simulink model "ThreeTankModelIITBombay"  (Simulink 6.6)
settings: Solver=ode3  StartTime=0.0  StopTime=2000  RelTol=1e-3
libraries: simulink3 x4
settings Model: Creator=nina  LastModifiedBy=nina
settings OptimizationCC: InlineInvariantSignals=on
settings DebuggingCC: SignalResolutionControl=TryResolveAllWithWarning  SolverPrmCheckMsg=none  InheritedTsInSrcMsg=none  MultiTaskDSMMsg=warning  MultiTaskCondExecSysMsg=none  StrictBusMsg=None
settings HardwareCC: TargetUnknown=on
settings RTWCC: IncludeERTFirstTime=on
settings STFCustomTargetCC: TargetFcnLib=ansi_tfl_tmw.mat  GenFloatMathFcnCalls=ANSI_C  MatFileLogging=on  SystemTargetFile=grt.tlc

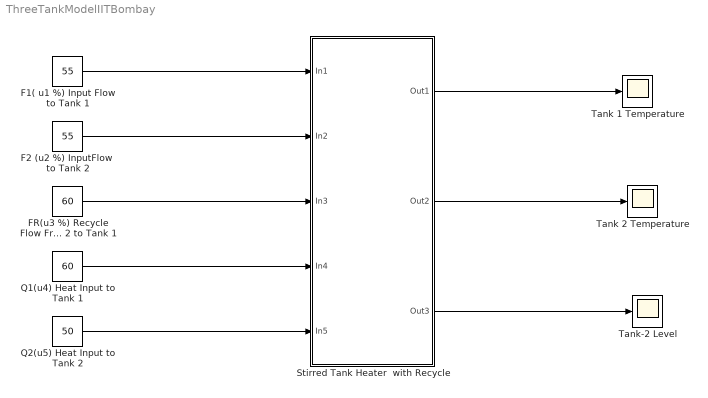
== system ThreeTankModelIITBombay ==
  "F1( u1 %) Input Flow to Tank 1 " : Constant  Value=55
  F2 (u2 %) InputFlow  to Tank 2 : Constant  Value=55
  FR(u3 %) Recycle Flow From Tank 2 to Tank 1 : Constant  Value=60
  Q1(u4) Heat Input to Tank 1 : Constant  Value=60
  Q2(u5) Heat Input to Tank 2 : Constant  Value=50
  "Stirred Tank Heater  with Recycle " : Subsystem
  Tank 1 Temperature : Scope
      settings: YMin=36.5  YMax=44.5  SaveName=ScopeData3  SampleInput=on  SampleTime=1
  Tank 2 Temperature : Scope
      settings: YMin=36.5  YMax=44.5  SampleInput=on  SampleTime=1
  Tank-2 Level : Scope
      settings: YMin=-2000  YMax=2000  SaveName=ScopeData2  SampleInput=on  SampleTime=1
  wires:
  "F1( u1 %) Input Flow to Tank 1 "/1 -> "Stirred Tank Heater  with Recycle "/1(In1)
  F2 (u2 %) InputFlow  to Tank 2/1 -> "Stirred Tank Heater  with Recycle "/2(In2)
  Q2(u5) Heat Input to Tank 2/1 -> "Stirred Tank Heater  with Recycle "/5(In5)
  "Stirred Tank Heater  with Recycle "/1(Out1) -> Tank 1 Temperature/1
  "Stirred Tank Heater  with Recycle "/3(Out3) -> Tank-2 Level/1
  FR(u3 %) Recycle Flow From Tank 2 to Tank 1/1 -> "Stirred Tank Heater  with Recycle "/3(In3)
  Q1(u4) Heat Input to Tank 1/1 -> "Stirred Tank Heater  with Recycle "/4(In4)
  "Stirred Tank Heater  with Recycle "/2(Out2) -> Tank 2 Temperature/1

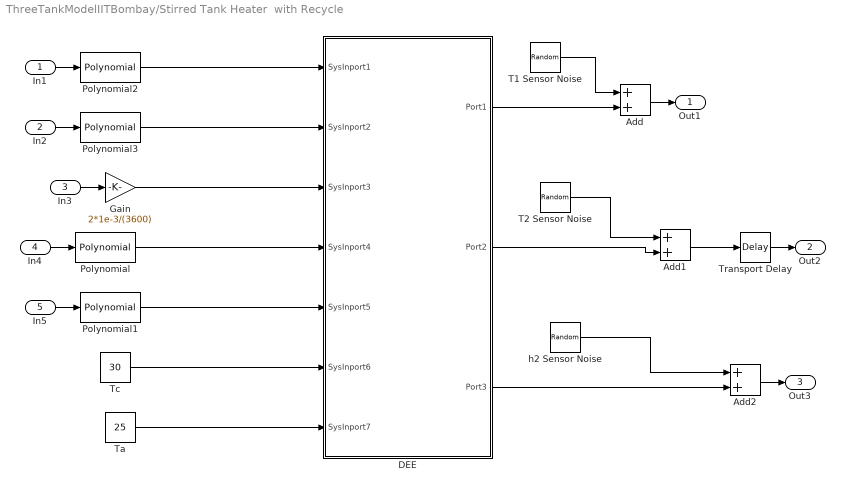
== system ThreeTankModelIITBombay/Stirred Tank Heater  with Recycle  ==
  In1 : Inport
  In2 : Inport  Port=2
  In3 : Inport  Port=3
  In4 : Inport  Port=4
  In5 : Inport  Port=5
  Add : Sum  InputSameDT=on
  Add1 : Sum  InputSameDT=on
  Add2 : Sum  InputSameDT=on
  DEE : Subsystem
      settings: OpenFcn=diffeqed
      mask Type: Differential Equation Editor (DEE)
      mask Display: disp('Modified STH')
  Gain : Gain  Gain=2*1e-3/(3600)
  Polynomial : simulink3/Functions & Tables/Polynomial  coefs="[ -0.0073  0.9893  7.9798 0]"
  Polynomial1 : simulink3/Functions & Tables/Polynomial  coefs=[ -0.008 +0.96 +14.4 104 ]
  Polynomial2 : simulink3/Functions & Tables/Polynomial  coefs="(1e-3/3600)*[ 0.00045  -0.034  2.2  -5.3 ]"
  Polynomial3 : simulink3/Functions & Tables/Polynomial  coefs="(1e-3/3600)*[  -0.00014  0.055  -1.8  77  ]"
  T1 Sensor Noise : RandomNumber  Variance=0.12^2
  T2 Sensor Noise : RandomNumber  Variance=0.15^2
  Ta : Constant  Value=25
  Tc : Constant  Value=30
  Transport Delay : TransportDelay  DelayTime=15  InitialOutput=4.690836960098364e+001
  h2 Sensor Noise : RandomNumber  Variance=0.015^2
  Out1 : Outport
  Out2 : Outport  Port=2
  Out3 : Outport  Port=3
  wires:
  Polynomial2/1 -> DEE/1(SysInport1)
  Tc/1 -> DEE/6(SysInport6)
  Polynomial3/1 -> DEE/2(SysInport2)
  Ta/1 -> DEE/7(SysInport7)
  Polynomial1/1 -> DEE/5(SysInport5)
  Polynomial/1 -> DEE/4(SysInport4)
  DEE/1(Port1) -> Add/2
  DEE/2(Port2) -> Add1/2
  DEE/3(Port3) -> Add2/2
  Add1/1 -> Transport Delay/1
  T1 Sensor Noise/1 -> Add/1
  Gain/1 -> DEE/3(SysInport3)
  T2 Sensor Noise/1 -> Add1/1
  h2 Sensor Noise/1 -> Add2/1
  In1/1 -> Polynomial2/1
  Add/1 -> Out1/1
  In2/1 -> Polynomial3/1
  In3/1 -> Gain/1
  In4/1 -> Polynomial/1
  Transport Delay/1 -> Out2/1
  In5/1 -> Polynomial1/1
  Add2/1 -> Out3/1

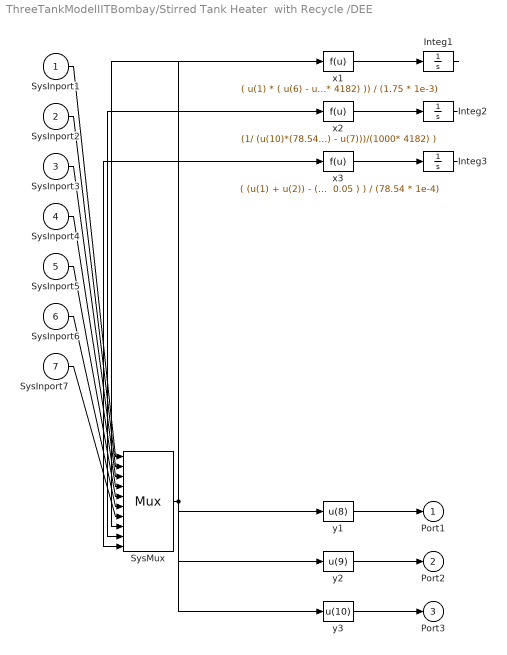
== system ThreeTankModelIITBombay/Stirred Tank Heater  with Recycle /DEE ==
  SysInport1 : Inport
  SysInport2 : Inport  Port=2
  SysInport3 : Inport  Port=3
  SysInport4 : Inport  Port=4
  SysInport5 : Inport  Port=5
  SysInport6 : Inport  Port=6
  SysInport7 : Inport  Port=7
  Integ1 : Integrator  InitialCondition=4.997718923518269e+001
  Integ2 : Integrator  InitialCondition=4.690836960098364e+001
  Integ3 : Integrator  InitialCondition=3.622745839296775e-001
  SysMux : Mux  Inputs=10
  x1 : Fcn  Expr=( u(1) * ( u(6) - u(8) ) + u(3) * (u(9) - u(8)) + ( u(4)/(1000* 4182) )) / (1.75 * 1e-3)
  x2 : Fcn  Expr=(1/ (u(10)*(78.54 * 1e-4))) * ( u(1)*(u(8) - u(9)) + u(2)*(u(6) -u(9)) - u(3)*(u(9) - u(8)) + ( u(5) - (2*pi*0.05*235.1043)*u(10)*(u(9) - u(7)))/(1000* 4182) )
  x3 : Fcn  Expr="( (u(1) + u(2)) - (0.1)*1e-3* sqrt( 10.35*u(10)^3- 9.39*u(10)^2+3.11*u(10) -  0.05 ) ) / (78.54 * 1e-4)"
  y1 : Fcn  Expr=u(8)
  y2 : Fcn  Expr=u(9)
  y3 : Fcn  Expr=u(10)
  Port1 : Outport
  Port2 : Outport  Port=2
  Port3 : Outport  Port=3
  wires:
  SysInport1/1 -> SysMux/1
  SysInport2/1 -> SysMux/2
  SysInport3/1 -> SysMux/3
  SysInport4/1 -> SysMux/4
  SysInport5/1 -> SysMux/5
  SysInport6/1 -> SysMux/6
  SysInport7/1 -> SysMux/7
  SysMux/1 -> x1/1, x2/1, x3/1, y1/1, y2/1, y3/1
  x1/1 -> Integ1/1
  Integ1/1 -> SysMux/8
  x2/1 -> Integ2/1
  Integ2/1 -> SysMux/9
  x3/1 -> Integ3/1
  Integ3/1 -> SysMux/10
  y1/1 -> Port1/1
  y2/1 -> Port2/1
  y3/1 -> Port3/1
